simulink model "Retro_Edo_2"  (Simulink 8.6)
settings: Solver=VariableStepAuto  StartTime=0.0  StopTime=10.0  RelTol=1e-3
values from neighbouring files (symbols this model uses):
  Id = eye(4)    [retro.m]
undefined symbols (not defined in the file or in its folder): A, b, f2, T2, vcero, x0
settings Model: Creator=Tlakatl  LastModifiedBy=Tlayekanketl
settings DebuggingCC: SolverPrmCheckMsg=none  FcnCallInpInsideContextMsg=EnableAllAsWarning
settings ConfigComp: CovSFcnEnable=off

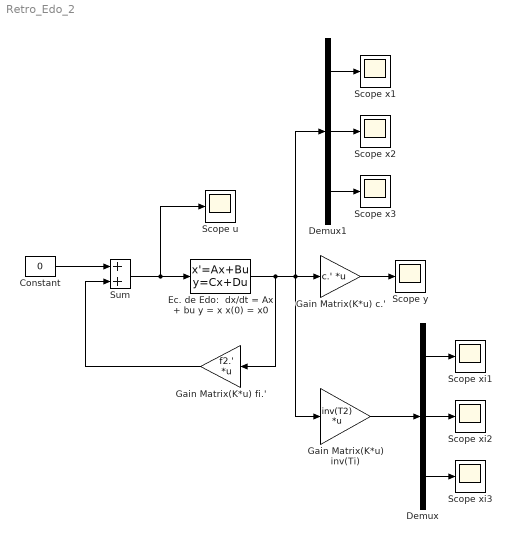
== system Retro_Edo_2 ==
  Constant : Constant  Value=0
  Demux : Demux  Outputs=3
  Demux1 : Demux  Outputs=3
  Ec. de Edo:  dx/dt = Ax + bu y = x x(0) = x0 : StateSpace  A=A  B=b  C=Id  D=vcero  X0=x0
  Gain Matrix(K*u) c.' : Gain  Gain=c.'  Multiplication=Matrix(K*u)
  Gain Matrix(K*u) fi.' : Gain  Gain=f2.'  Multiplication=Matrix(K*u) (u vector)
  Gain Matrix(K*u) inv(Ti) : Gain  Gain=inv(T2)  Multiplication=Matrix(K*u)
  Scope u : Scope
  Scope x1 : Scope
  Scope x2 : Scope
  Scope x3 : Scope
  Scope xi1 : Scope
  Scope xi2 : Scope
  Scope xi3 : Scope
  Scope y : Scope
  Sum : Sum
  wires:
  Sum/1 -> Ec. de Edo:  dx/dt = Ax + bu y = x x(0) = x0/1, Scope u/1
  Ec. de Edo:  dx/dt = Ax + bu y = x x(0) = x0/1 -> Gain Matrix(K*u) fi.'/1, Gain Matrix(K*u) c.'/1, Gain Matrix(K*u) inv(Ti)/1, Demux1/1
  Gain Matrix(K*u) fi.'/1 -> Sum/2
  Constant/1 -> Sum/1
  Gain Matrix(K*u) c.'/1 -> Scope y/1
  Gain Matrix(K*u) inv(Ti)/1 -> Demux/1
  Demux/3 -> Scope xi3/1
  Demux/2 -> Scope xi2/1
  Demux/1 -> Scope xi1/1
  Demux1/3 -> Scope x3/1
  Demux1/2 -> Scope x2/1
  Demux1/1 -> Scope x1/1
